simulink model "Send"  (R2017b)
settings: Solver=VariableStepAuto  StartTime=0.0  StopTime=inf  RelTol=1e-3
undefined symbols (not defined in the file or in its folder): serial
libraries: instrumentlib x2
settings Model: Creator=CIRA  LastModifiedBy=CIRA

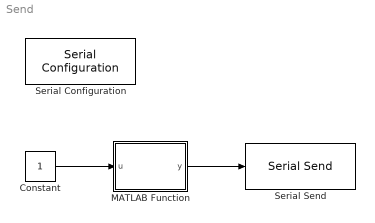
== system Send ==
  Constant : Constant
  MATLAB Function : MATLAB Function  TreatAsAtomicUnit=on
  Serial Configuration : instrumentlib/Serial Configuration  Priority=-200000  ComPortMenu=COM6  ComPort=COM6  ObjConstructor=serial('COM6');  BaudRate=9600  DataBits=8  Parity=none  StopBits=1  FlowControl=none  Timeout=10  ByteOrder=LittleEndian
  Serial Send : instrumentlib/Serial Send  ComPortMenu=COM6  ComPort=COM6  ObjConstructor=serial('COM6');  Terminator='%'  EnableBlockingMode=on
  wires:
  MATLAB Function/1(y) -> Serial Send/1
  Constant/1 -> MATLAB Function/1(u)

== matlab function Send/MATLAB Function ==
  data: u input; y output
function y = fcn(u)
if u == 1

puerto=serial('COM6');
puerto.BaudRate=19200;
fopen(puerto); %el puerto a utilizar
writeline(puerto,"AXEL")
configureTerminator(puerto,"%")
 %cierra y borra el puerto utilizado, borra todas las variables utilizadas
 fclose (puerto) ;
 delete (puerto) ;
end
y = u;
